simulink model "Wind_Model"  (R2025b)
settings: Solver=VariableStepAuto  StartTime=0.0  StopTime=10.0  RelTol=1e-3
values from neighbouring files (symbols this model uses):
  q = MX.sym('q', 4)    [CasADiDynamics.m]    (also in FlightDynamicsGen.m = [q0; q1; q2; q3])
  r = MX.sym('r', 3)    [CasADiDynamics.m]    (also in FlightDynamicsGen.m = [r1; r2; r3])
undefined symbols (not defined in the file or in its folder): constantsASTRA, dt_SIM, F, Light, MIL, windMerid, windZonal
libraries: aerolibwind2 x1
settings Model: Creator=andrew  LastModifiedBy=andrew

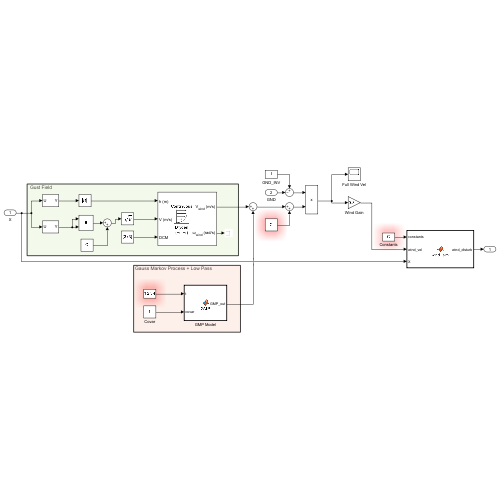
[thumbnail: Simulink's stored preview of the top-level diagram]
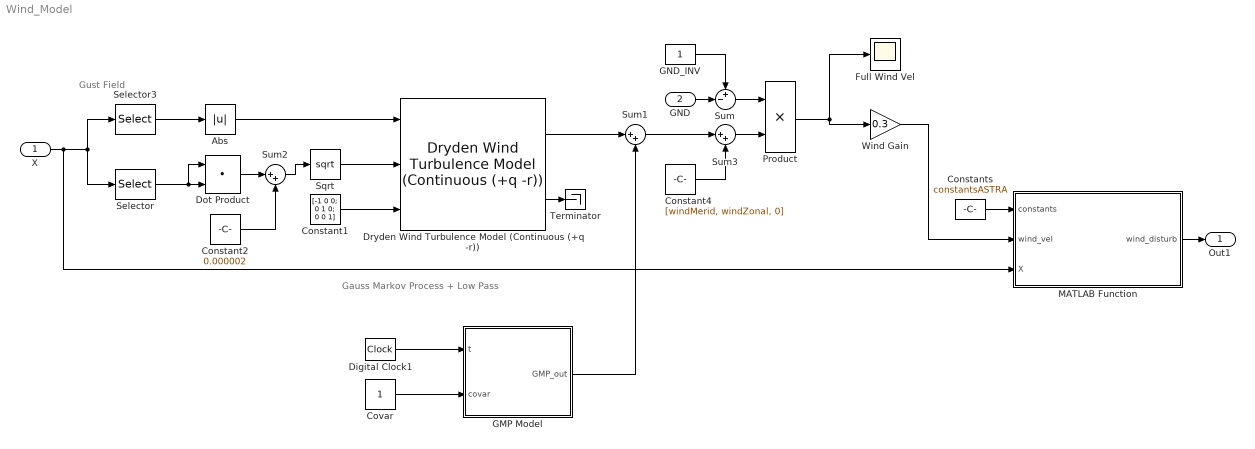
== system Wind_Model ==
  note: Gust Field
  note: Gauss Markov Process + Low Pass
  X : Inport
  GND : Inport  Port=2
  Abs : Abs  SaturateOnIntegerOverflow=off
  Constant1 : Constant  Value=[-1 0 0; 0 1 0; 0 0 1]
  Constant2 : Constant  Value=0.000002
  Constant4 : Constant  Value=[windMerid, windZonal, 0]
  Constants : Constant  Value=constantsASTRA  OutDataTypeStr=Bus: slBus1
  Covar : Constant
  Digital Clock1 : DigitalClock  SampleTime=dt_SIM
  Dot Product : DotProduct  OutDataTypeStr=Inherit: Inherit via internal rule
  Dryden Wind Turbulence Model (Continuous (+q -r)) : aerolibwind2/Dryden Wind Turbulence Model  (Continuous (+q -r))  units=Metric (MKS)  spec=MIL-F-8785C  model=Continuous Dryden (+q +r)  W20=15  Wdeg=0  TurbProb=10^-2 - Light  L_high=533.4  Wingspan=10  ts=0.1  Seed=[23341 23342 23343 23344]  T_on=on
  Full Wind Vel : Scope
      settings: ActiveDisplayYMinimum=-5.4482795847516687  ActiveDisplayYMaximum=3.7310351492092773  DataLoggingVariableName=ScopeData13
  GMP Model : MATLAB Function  TreatAsAtomicUnit=on
  GND_INV : Constant
  MATLAB Function : MATLAB Function  TreatAsAtomicUnit=on
  Product : Product
  Selector : Selector  InputPortWidth=16  IndexOptions=Index vector (dialog)  Indices=[8:10]  OutputSizes=1
  Selector3 : Selector  InputPortWidth=16  IndexOptions=Index vector (dialog)  Indices=7  OutputSizes=1
  Sqrt : Sqrt
  Sum : Sum  Inputs=+-|
  Sum1 : Sum  Inputs=|++
  Sum2 : Sum  Inputs=|++
  Sum3 : Sum  Inputs=|++
  Terminator : Terminator
  Wind Gain : Gain  Gain=0.3
  Out1 : Outport
  wires:
  Sqrt/1 -> Dryden Wind Turbulence Model (Continuous (+q -r))/2
  Sum2/1 -> Sqrt/1
  Constant1/1 -> Dryden Wind Turbulence Model (Continuous (+q -r))/3
  Dryden Wind Turbulence Model (Continuous (+q -r))/2 -> Terminator/1
  X/1 -> MATLAB Function/3(X), Selector3/1, Selector/1
  Selector/1 -> Dot Product/1, Dot Product/2
  Dot Product/1 -> Sum2/1
  Constant2/1 -> Sum2/2
  Abs/1 -> Dryden Wind Turbulence Model (Continuous (+q -r))/1
  Selector3/1 -> Abs/1
  Covar/1 -> GMP Model/2(covar)
  Digital Clock1/1 -> GMP Model/1(t)
  GND/1 -> Sum/2
  GND_INV/1 -> Sum/1
  Sum/1 -> Product/1
  Dryden Wind Turbulence Model (Continuous (+q -r))/1 -> Sum1/1
  GMP Model/1(GMP_out) -> Sum1/2
  Sum1/1 -> Sum3/1
  Constant4/1 -> Sum3/2
  Product/1 -> Full Wind Vel/1, Wind Gain/1
  Sum3/1 -> Product/2
  Wind Gain/1 -> MATLAB Function/2(wind_vel)
  Constants/1 -> MATLAB Function/1(constants)
  MATLAB Function/1(wind_disturb) -> Out1/1

== matlab function Wind_Model/GMP Model ==
  data: t input; GMP_out output; covar input
function GMP_out = GMP(t, covar)

persistent errorval lastTime EMA
if isempty(errorval)
    errorval = 0;
    EMA = 0;
    lastTime = 0;  % Update last timestamp
end

dT = t - lastTime;

% First order Gauss Markov Process for additional disturbance
decay = 10;
beta = exp(-dT / decay);
errorval = beta * errorval + sqrt(1 - beta^2) * covar * randn;

% EMA Step to kill High Freq. Noise
EMA = ExpMovingAvg(errorval, EMA, 0.05);
GMP_out = EMA * ones(3,1);
lastTime = t;

== matlab function Wind_Model/MATLAB Function ==
  data: constants input; wind_vel input; X input; wind_disturb output
function wind_disturb = wind_sim(constants, wind_vel, X)

wind_disturb = wind(constants, wind_vel, X);
